simulink model "FDIA_21_TRAINING"  (R2021a)
settings: Solver=ode113  StartTime=0.0  StopTime=20  RelTol=1e-3
undefined symbols (not defined in the file or in its folder): Discrete, linsys1, Time
libraries: spsThreePhaseVIMeasurementLib x46, spsThreePhasePISectionLineLib x20, spsThreePhaseSeriesRLCLoadLib x12, simulink x6, spsThreePhaseTransformerTwoWindingsLib x5, spsThreePhaseBreakerLib x5, ctrlSharedLib x3, spsThreePhaseDynamicLoadLib x3, spsSynchronousMachinepuStandardLib x3, spsThreePhaseParallelRLCLoadLib x3, spsExcitationSystemLib x3, spsGenericPowerSystemStabilizerLib x3
(part 3 of 3)

== system FDIA_21_TRAINING/Subsystem1/Bus_1 ==
  Three-Phase V-I Measurement : spsThreePhaseVIMeasurementLib/Three-Phase V-I Measurement  VoltageMeasurement=phase-to-phase  SetLabelV=on  LabelV=VB_1  Vpu=off  VpuLL=off  CurrentMeasurement=yes  SetLabelI=on  LabelI=IB_1  Ipu=off  Pbase=100e6  Vbase=500e3  OutputType=Complex  PhasorSimulation=off  PSBequivalent=0
  Three-Phase V-I Measurement1 : spsThreePhaseVIMeasurementLib/Three-Phase V-I Measurement  VoltageMeasurement=phase-to-phase  SetLabelV=on  LabelV=V_B1  Vpu=off  VpuLL=off  CurrentMeasurement=yes  SetLabelI=on  LabelI=I_B1  Ipu=off  Pbase=100e6  Vbase=500e3  OutputType=Complex  PhasorSimulation=off  PSBequivalent=0
  Conn1 : PMIOPort  Side=Left
  Conn2 : PMIOPort  Port=2  Side=Right
  Conn3 : PMIOPort  Port=3  Side=Left
  Conn4 : PMIOPort  Port=4  Side=Right
  Conn5 : PMIOPort  Port=5  Side=Right
  Conn6 : PMIOPort  Port=6  Side=Left
  Conn7 : PMIOPort  Port=7  Side=Right
  Conn8 : PMIOPort  Port=8  Side=Right
  Conn9 : PMIOPort  Port=9  Side=Right
  connections:
  Conn6/RConn1 -- Three-Phase V-I Measurement1/LConn1 -- Three-Phase V-I Measurement/LConn3
  Three-Phase V-I Measurement/RConn2 -- Conn4/RConn1
  Three-Phase V-I Measurement1/RConn2 -- Conn8/RConn1
  Conn3/RConn1 -- Three-Phase V-I Measurement1/LConn2 -- Three-Phase V-I Measurement/LConn2
  Conn1/RConn1 -- Three-Phase V-I Measurement1/LConn3 -- Three-Phase V-I Measurement/LConn1
  Three-Phase V-I Measurement/RConn1 -- Conn5/RConn1
  Three-Phase V-I Measurement/RConn3 -- Conn2/RConn1
  Three-Phase V-I Measurement1/RConn1 -- Conn9/RConn1
  Three-Phase V-I Measurement1/RConn3 -- Conn7/RConn1

== system FDIA_21_TRAINING/Subsystem1/Bus_10 ==
  Three-Phase V-I Measurement : spsThreePhaseVIMeasurementLib/Three-Phase V-I Measurement  VoltageMeasurement=phase-to-phase  SetLabelV=on  LabelV=VB_10  Vpu=off  VpuLL=off  CurrentMeasurement=yes  SetLabelI=on  LabelI=IB_10  Ipu=off  Pbase=100e6  Vbase=500e3  OutputType=Complex  PhasorSimulation=off  PSBequivalent=0
  Three-Phase V-I Measurement1 : spsThreePhaseVIMeasurementLib/Three-Phase V-I Measurement  VoltageMeasurement=phase-to-phase  SetLabelV=on  LabelV=V_B10  Vpu=off  VpuLL=off  CurrentMeasurement=yes  SetLabelI=on  LabelI=I_B10  Ipu=off  Pbase=100e6  Vbase=500e3  OutputType=Complex  PhasorSimulation=off  PSBequivalent=0
  Conn1 : PMIOPort  Side=Left
  Conn2 : PMIOPort  Port=2  Side=Right
  Conn3 : PMIOPort  Port=3  Side=Left
  Conn4 : PMIOPort  Port=4  Side=Right
  Conn5 : PMIOPort  Port=5  Side=Right
  Conn6 : PMIOPort  Port=6  Side=Left
  Conn7 : PMIOPort  Port=7  Side=Right
  Conn8 : PMIOPort  Port=8  Side=Right
  Conn9 : PMIOPort  Port=9  Side=Right
  connections:
  Conn1/RConn1 -- Three-Phase V-I Measurement1/LConn3 -- Three-Phase V-I Measurement/LConn1
  Conn3/RConn1 -- Three-Phase V-I Measurement1/LConn2 -- Three-Phase V-I Measurement/LConn2
  Conn8/RConn1 -- Three-Phase V-I Measurement1/RConn2
  Three-Phase V-I Measurement/RConn2 -- Conn4/RConn1
  Conn6/RConn1 -- Three-Phase V-I Measurement1/LConn1 -- Three-Phase V-I Measurement/LConn3
  Conn7/RConn1 -- Three-Phase V-I Measurement1/RConn1
  Conn9/RConn1 -- Three-Phase V-I Measurement1/RConn3
  Conn2/RConn1 -- Three-Phase V-I Measurement/RConn1
  Conn5/RConn1 -- Three-Phase V-I Measurement/RConn3

== system FDIA_21_TRAINING/Subsystem1/Bus_11 ==
  Three-Phase V-I Measurement : spsThreePhaseVIMeasurementLib/Three-Phase V-I Measurement  VoltageMeasurement=phase-to-phase  SetLabelV=on  LabelV=VB_11  Vpu=off  VpuLL=off  CurrentMeasurement=yes  SetLabelI=on  LabelI=IB_11  Ipu=off  Pbase=100e6  Vbase=500e3  OutputType=Complex  PhasorSimulation=off  PSBequivalent=0
  Three-Phase V-I Measurement1 : spsThreePhaseVIMeasurementLib/Three-Phase V-I Measurement  VoltageMeasurement=phase-to-phase  SetLabelV=on  LabelV=V_B11  Vpu=off  VpuLL=off  CurrentMeasurement=yes  SetLabelI=on  LabelI=I_B11  Ipu=off  Pbase=100e6  Vbase=500e3  OutputType=Complex  PhasorSimulation=off  PSBequivalent=0
  Conn1 : PMIOPort  Side=Left
  Conn2 : PMIOPort  Port=2  Side=Right
  Conn3 : PMIOPort  Port=3  Side=Left
  Conn4 : PMIOPort  Port=4  Side=Right
  Conn5 : PMIOPort  Port=5  Side=Right
  Conn6 : PMIOPort  Port=6  Side=Left
  Conn7 : PMIOPort  Port=7  Side=Right
  Conn8 : PMIOPort  Port=8  Side=Right
  Conn9 : PMIOPort  Port=9  Side=Right
  connections:
  Three-Phase V-I Measurement/RConn3 -- Conn5/RConn1
  Three-Phase V-I Measurement/RConn1 -- Conn2/RConn1
  Three-Phase V-I Measurement1/RConn3 -- Conn9/RConn1
  Three-Phase V-I Measurement1/RConn1 -- Conn7/RConn1
  Conn6/RConn1 -- Three-Phase V-I Measurement1/LConn1 -- Three-Phase V-I Measurement/LConn3
  Three-Phase V-I Measurement/RConn2 -- Conn4/RConn1
  Three-Phase V-I Measurement1/RConn2 -- Conn8/RConn1
  Conn3/RConn1 -- Three-Phase V-I Measurement1/LConn2 -- Three-Phase V-I Measurement/LConn2
  Conn1/RConn1 -- Three-Phase V-I Measurement1/LConn3 -- Three-Phase V-I Measurement/LConn1

== system FDIA_21_TRAINING/Subsystem1/Bus_12 ==
  Three-Phase V-I Measurement : spsThreePhaseVIMeasurementLib/Three-Phase V-I Measurement  VoltageMeasurement=phase-to-phase  SetLabelV=on  LabelV=VB_12  Vpu=off  VpuLL=off  CurrentMeasurement=yes  SetLabelI=on  LabelI=IB_12  Ipu=off  Pbase=100e6  Vbase=500e3  OutputType=Complex  PhasorSimulation=off  PSBequivalent=0
  Three-Phase V-I Measurement1 : spsThreePhaseVIMeasurementLib/Three-Phase V-I Measurement  VoltageMeasurement=phase-to-phase  SetLabelV=on  LabelV=V_B12  Vpu=off  VpuLL=off  CurrentMeasurement=yes  SetLabelI=on  LabelI=I_B12  Ipu=off  Pbase=100e6  Vbase=500e3  OutputType=Complex  PhasorSimulation=off  PSBequivalent=0
  Conn1 : PMIOPort  Side=Left
  Conn2 : PMIOPort  Port=2  Side=Right
  Conn3 : PMIOPort  Port=3  Side=Left
  Conn4 : PMIOPort  Port=4  Side=Right
  Conn5 : PMIOPort  Port=5  Side=Right
  Conn6 : PMIOPort  Port=6  Side=Left
  Conn7 : PMIOPort  Port=7  Side=Right
  Conn8 : PMIOPort  Port=8  Side=Right
  Conn9 : PMIOPort  Port=9  Side=Right
  connections:
  Conn1/RConn1 -- Three-Phase V-I Measurement1/LConn3 -- Three-Phase V-I Measurement/LConn1
  Conn3/RConn1 -- Three-Phase V-I Measurement1/LConn2 -- Three-Phase V-I Measurement/LConn2
  Three-Phase V-I Measurement1/RConn2 -- Conn8/RConn1
  Conn4/RConn1 -- Three-Phase V-I Measurement/RConn2
  Conn6/RConn1 -- Three-Phase V-I Measurement1/LConn1 -- Three-Phase V-I Measurement/LConn3
  Three-Phase V-I Measurement1/RConn1 -- Conn7/RConn1
  Three-Phase V-I Measurement1/RConn3 -- Conn9/RConn1
  Conn2/RConn1 -- Three-Phase V-I Measurement/RConn1
  Conn5/RConn1 -- Three-Phase V-I Measurement/RConn3

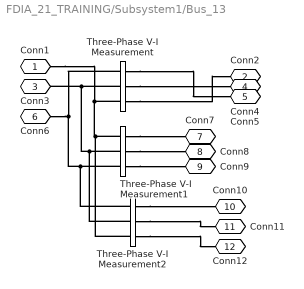
== system FDIA_21_TRAINING/Subsystem1/Bus_13 ==
  Three-Phase V-I Measurement : spsThreePhaseVIMeasurementLib/Three-Phase V-I Measurement  VoltageMeasurement=phase-to-phase  SetLabelV=on  LabelV=VB_13  Vpu=off  VpuLL=off  CurrentMeasurement=yes  SetLabelI=on  LabelI=IB_13  Ipu=off  Pbase=100e6  Vbase=500e3  OutputType=Complex  PhasorSimulation=off  PSBequivalent=0
  Three-Phase V-I Measurement1 : spsThreePhaseVIMeasurementLib/Three-Phase V-I Measurement  VoltageMeasurement=phase-to-phase  SetLabelV=on  LabelV=V_B13_13  Vpu=off  VpuLL=off  CurrentMeasurement=yes  SetLabelI=on  LabelI=I_B13_13  Ipu=off  Pbase=100e6  Vbase=500e3  OutputType=Complex  PhasorSimulation=off  PSBequivalent=0
  Three-Phase V-I Measurement2 : spsThreePhaseVIMeasurementLib/Three-Phase V-I Measurement  VoltageMeasurement=phase-to-phase  SetLabelV=on  LabelV=V_B13  Vpu=off  VpuLL=off  CurrentMeasurement=yes  SetLabelI=on  LabelI=I_B13  Ipu=off  Pbase=100e6  Vbase=500e3  OutputType=Complex  PhasorSimulation=off  PSBequivalent=0
  Conn1 : PMIOPort  Side=Left
  Conn2 : PMIOPort  Port=2  Side=Right
  Conn3 : PMIOPort  Port=3  Side=Left
  Conn4 : PMIOPort  Port=4  Side=Right
  Conn5 : PMIOPort  Port=5  Side=Right
  Conn6 : PMIOPort  Port=6  Side=Left
  Conn7 : PMIOPort  Port=7  Side=Right
  Conn8 : PMIOPort  Port=8  Side=Right
  Conn9 : PMIOPort  Port=9  Side=Right
  Conn10 : PMIOPort  Port=10  Side=Right
  Conn11 : PMIOPort  Port=11  Side=Right
  Conn12 : PMIOPort  Port=12  Side=Right
  connections:
  Three-Phase V-I Measurement2/LConn1 -- Three-Phase V-I Measurement1/LConn3 -- Three-Phase V-I Measurement/LConn1 -- Conn6/RConn1
  Conn3/RConn1 -- Three-Phase V-I Measurement/LConn2 -- Three-Phase V-I Measurement2/LConn2 -- Three-Phase V-I Measurement1/LConn2
  Three-Phase V-I Measurement1/RConn2 -- Conn8/RConn1
  Three-Phase V-I Measurement/RConn2 -- Conn4/RConn1
  Three-Phase V-I Measurement2/LConn3 -- Three-Phase V-I Measurement1/LConn1 -- Three-Phase V-I Measurement/LConn3 -- Conn1/RConn1
  Three-Phase V-I Measurement1/RConn1 -- Conn7/RConn1
  Three-Phase V-I Measurement1/RConn3 -- Conn9/RConn1
  Three-Phase V-I Measurement2/RConn1 -- Conn10/RConn1
  Three-Phase V-I Measurement2/RConn2 -- Conn11/RConn1
  Three-Phase V-I Measurement2/RConn3 -- Conn12/RConn1
  Three-Phase V-I Measurement/RConn1 -- Conn5/RConn1
  Three-Phase V-I Measurement/RConn3 -- Conn2/RConn1

== system FDIA_21_TRAINING/Subsystem1/Bus_14 ==
  Three-Phase V-I Measurement : spsThreePhaseVIMeasurementLib/Three-Phase V-I Measurement  VoltageMeasurement=phase-to-phase  SetLabelV=on  LabelV=VB_14  Vpu=off  VpuLL=off  CurrentMeasurement=yes  SetLabelI=on  LabelI=IB_14  Ipu=off  Pbase=100e6  Vbase=500e3  OutputType=Complex  PhasorSimulation=off  PSBequivalent=0
  Three-Phase V-I Measurement1 : spsThreePhaseVIMeasurementLib/Three-Phase V-I Measurement  VoltageMeasurement=phase-to-phase  SetLabelV=on  LabelV=V_B14  Vpu=off  VpuLL=off  CurrentMeasurement=yes  SetLabelI=on  LabelI=I_B14  Ipu=off  Pbase=100e6  Vbase=500e3  OutputType=Complex  PhasorSimulation=off  PSBequivalent=0
  Conn1 : PMIOPort  Side=Left
  Conn2 : PMIOPort  Port=2  Side=Right
  Conn3 : PMIOPort  Port=3  Side=Left
  Conn4 : PMIOPort  Port=4  Side=Right
  Conn5 : PMIOPort  Port=5  Side=Right
  Conn6 : PMIOPort  Port=6  Side=Left
  Conn7 : PMIOPort  Port=7  Side=Right
  Conn8 : PMIOPort  Port=8  Side=Right
  Conn9 : PMIOPort  Port=9  Side=Right
  connections:
  Conn1/RConn1 -- Three-Phase V-I Measurement1/LConn3 -- Three-Phase V-I Measurement/LConn1
  Conn3/RConn1 -- Three-Phase V-I Measurement1/LConn2 -- Three-Phase V-I Measurement/LConn2
  Three-Phase V-I Measurement1/RConn2 -- Conn8/RConn1
  Three-Phase V-I Measurement/RConn2 -- Conn4/RConn1
  Conn6/RConn1 -- Three-Phase V-I Measurement1/LConn1 -- Three-Phase V-I Measurement/LConn3
  Three-Phase V-I Measurement/RConn1 -- Conn2/RConn1
  Three-Phase V-I Measurement/RConn3 -- Conn5/RConn1
  Three-Phase V-I Measurement1/RConn3 -- Conn7/RConn1
  Three-Phase V-I Measurement1/RConn1 -- Conn9/RConn1

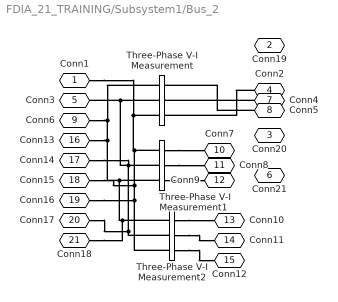
== system FDIA_21_TRAINING/Subsystem1/Bus_2 ==
  Three-Phase V-I Measurement : spsThreePhaseVIMeasurementLib/Three-Phase V-I Measurement  VoltageMeasurement=phase-to-phase  SetLabelV=on  LabelV=VB_2  Vpu=off  VpuLL=off  CurrentMeasurement=yes  SetLabelI=on  LabelI=IB_2  Ipu=off  Pbase=100e6  Vbase=500e3  OutputType=Complex  PhasorSimulation=off  PSBequivalent=0
  Three-Phase V-I Measurement1 : spsThreePhaseVIMeasurementLib/Three-Phase V-I Measurement  VoltageMeasurement=phase-to-phase  SetLabelV=on  LabelV=V_B22  Vpu=off  VpuLL=off  CurrentMeasurement=yes  SetLabelI=on  LabelI=I_B22  Ipu=off  Pbase=100e6  Vbase=500e3  OutputType=Complex  PhasorSimulation=off  PSBequivalent=0
  Three-Phase V-I Measurement2 : spsThreePhaseVIMeasurementLib/Three-Phase V-I Measurement  VoltageMeasurement=phase-to-phase  SetLabelV=on  LabelV=V_B2  Vpu=off  VpuLL=off  CurrentMeasurement=yes  SetLabelI=on  LabelI=I_B2  Ipu=off  Pbase=100e6  Vbase=500e3  OutputType=Complex  PhasorSimulation=off  PSBequivalent=0
  Conn1 : PMIOPort  Side=Left
  Conn19 : PMIOPort  Port=2  Side=Right
  Conn20 : PMIOPort  Port=3  Side=Right
  Conn2 : PMIOPort  Port=4  Side=Right
  Conn3 : PMIOPort  Port=5  Side=Left
  Conn21 : PMIOPort  Port=6  Side=Right
  Conn4 : PMIOPort  Port=7  Side=Right
  Conn5 : PMIOPort  Port=8  Side=Right
  Conn6 : PMIOPort  Port=9  Side=Left
  Conn7 : PMIOPort  Port=10  Side=Right
  Conn8 : PMIOPort  Port=11  Side=Right
  Conn9 : PMIOPort  Port=12  Side=Right
  Conn10 : PMIOPort  Port=13  Side=Right
  Conn11 : PMIOPort  Port=14  Side=Right
  Conn12 : PMIOPort  Port=15  Side=Right
  Conn13 : PMIOPort  Port=16  Side=Left
  Conn14 : PMIOPort  Port=17  Side=Left
  Conn15 : PMIOPort  Port=18  Side=Left
  Conn16 : PMIOPort  Port=19  Side=Left
  Conn17 : PMIOPort  Port=20  Side=Left
  Conn18 : PMIOPort  Port=21  Side=Left
  connections:
  Conn18/RConn1 -- Three-Phase V-I Measurement2/LConn1 -- Three-Phase V-I Measurement1/LConn3 -- Conn13/RConn1 -- Three-Phase V-I Measurement/LConn1 -- Conn6/RConn1
  Conn3/RConn1 -- Three-Phase V-I Measurement/LConn2 -- Three-Phase V-I Measurement1/LConn2 -- Three-Phase V-I Measurement2/LConn2 -- Conn17/RConn1 -- Conn14/RConn1
  Three-Phase V-I Measurement1/RConn2 -- Conn8/RConn1
  Conn4/RConn1 -- Three-Phase V-I Measurement/RConn2
  Conn16/RConn1 -- Three-Phase V-I Measurement2/LConn3 -- Conn15/RConn1 -- Three-Phase V-I Measurement1/LConn1 -- Three-Phase V-I Measurement/LConn3 -- Conn1/RConn1
  Three-Phase V-I Measurement1/RConn1 -- Conn7/RConn1
  Three-Phase V-I Measurement1/RConn3 -- Conn9/RConn1
  Three-Phase V-I Measurement2/RConn1 -- Conn10/RConn1
  Three-Phase V-I Measurement2/RConn2 -- Conn11/RConn1
  Three-Phase V-I Measurement2/RConn3 -- Conn12/RConn1
  Conn5/RConn1 -- Three-Phase V-I Measurement/RConn1
  Conn2/RConn1 -- Three-Phase V-I Measurement/RConn3

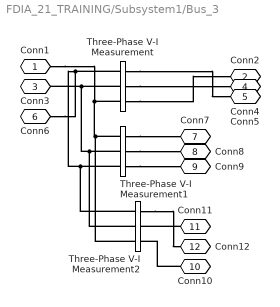
== system FDIA_21_TRAINING/Subsystem1/Bus_3 ==
  Three-Phase V-I Measurement : spsThreePhaseVIMeasurementLib/Three-Phase V-I Measurement  VoltageMeasurement=phase-to-phase  SetLabelV=on  LabelV=VB_3  Vpu=off  VpuLL=off  CurrentMeasurement=yes  SetLabelI=on  LabelI=IB_3  Ipu=off  Pbase=100e6  Vbase=500e3  OutputType=Complex  PhasorSimulation=off  PSBequivalent=0
  Three-Phase V-I Measurement1 : spsThreePhaseVIMeasurementLib/Three-Phase V-I Measurement  VoltageMeasurement=phase-to-phase  SetLabelV=on  LabelV=V_B33  Vpu=off  VpuLL=off  CurrentMeasurement=yes  SetLabelI=on  LabelI=I_B33  Ipu=off  Pbase=100e6  Vbase=500e3  OutputType=Complex  PhasorSimulation=off  PSBequivalent=0
  Three-Phase V-I Measurement2 : spsThreePhaseVIMeasurementLib/Three-Phase V-I Measurement  VoltageMeasurement=phase-to-phase  SetLabelV=on  LabelV=V_B3  Vpu=off  VpuLL=off  CurrentMeasurement=yes  SetLabelI=on  LabelI=I_B3  Ipu=off  Pbase=100e6  Vbase=500e3  OutputType=Complex  PhasorSimulation=off  PSBequivalent=0
  Conn1 : PMIOPort  Side=Left
  Conn2 : PMIOPort  Port=2  Side=Right
  Conn3 : PMIOPort  Port=3  Side=Left
  Conn4 : PMIOPort  Port=4  Side=Right
  Conn5 : PMIOPort  Port=5  Side=Right
  Conn6 : PMIOPort  Port=6  Side=Left
  Conn7 : PMIOPort  Port=7  Side=Right
  Conn8 : PMIOPort  Port=8  Side=Right
  Conn9 : PMIOPort  Port=9  Side=Right
  Conn10 : PMIOPort  Port=10  Side=Right
  Conn11 : PMIOPort  Port=11  Side=Right
  Conn12 : PMIOPort  Port=12  Side=Right
  connections:
  Conn11/RConn1 -- Three-Phase V-I Measurement2/RConn2
  Three-Phase V-I Measurement1/RConn3 -- Conn9/RConn1
  Three-Phase V-I Measurement1/RConn1 -- Conn7/RConn1
  Three-Phase V-I Measurement2/LConn3 -- Three-Phase V-I Measurement1/LConn1 -- Three-Phase V-I Measurement/LConn3 -- Conn1/RConn1
  Three-Phase V-I Measurement/RConn2 -- Conn4/RConn1
  Three-Phase V-I Measurement1/RConn2 -- Conn8/RConn1
  Three-Phase V-I Measurement2/LConn2 -- Three-Phase V-I Measurement1/LConn2 -- Three-Phase V-I Measurement/LConn2 -- Conn3/RConn1
  Three-Phase V-I Measurement2/LConn1 -- Three-Phase V-I Measurement1/LConn3 -- Three-Phase V-I Measurement/LConn1 -- Conn6/RConn1
  Conn10/RConn1 -- Three-Phase V-I Measurement2/RConn3
  Three-Phase V-I Measurement2/RConn1 -- Conn12/RConn1
  Three-Phase V-I Measurement/RConn3 -- Conn2/RConn1
  Three-Phase V-I Measurement/RConn1 -- Conn5/RConn1

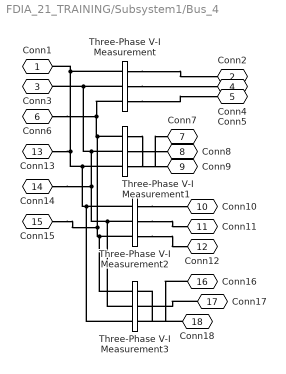
== system FDIA_21_TRAINING/Subsystem1/Bus_4 ==
  Three-Phase V-I Measurement : spsThreePhaseVIMeasurementLib/Three-Phase V-I Measurement  VoltageMeasurement=phase-to-phase  SetLabelV=on  LabelV=VB_4  Vpu=off  VpuLL=off  CurrentMeasurement=yes  SetLabelI=on  LabelI=IB_4  Ipu=off  Pbase=100e6  Vbase=500e3  OutputType=Complex  PhasorSimulation=off  PSBequivalent=0
  Three-Phase V-I Measurement1 : spsThreePhaseVIMeasurementLib/Three-Phase V-I Measurement  VoltageMeasurement=phase-to-phase  SetLabelV=on  LabelV=V_B44  Vpu=off  VpuLL=off  CurrentMeasurement=yes  SetLabelI=on  LabelI=I_B44  Ipu=off  Pbase=100e6  Vbase=500e3  OutputType=Complex  PhasorSimulation=off  PSBequivalent=0
  Three-Phase V-I Measurement2 : spsThreePhaseVIMeasurementLib/Three-Phase V-I Measurement  VoltageMeasurement=phase-to-phase  SetLabelV=on  LabelV=V_B4  Vpu=off  VpuLL=off  CurrentMeasurement=yes  SetLabelI=on  LabelI=I_B4  Ipu=off  Pbase=100e6  Vbase=500e3  OutputType=Complex  PhasorSimulation=off  PSBequivalent=0
  Three-Phase V-I Measurement3 : spsThreePhaseVIMeasurementLib/Three-Phase V-I Measurement  VoltageMeasurement=phase-to-phase  SetLabelV=on  LabelV=V_B4_4  Vpu=off  VpuLL=off  CurrentMeasurement=yes  SetLabelI=on  LabelI=I_B4_4  Ipu=off  Pbase=100e6  Vbase=500e3  OutputType=Complex  PhasorSimulation=off  PSBequivalent=0
  Conn1 : PMIOPort  Side=Left
  Conn2 : PMIOPort  Port=2  Side=Right
  Conn3 : PMIOPort  Port=3  Side=Left
  Conn4 : PMIOPort  Port=4  Side=Right
  Conn5 : PMIOPort  Port=5  Side=Right
  Conn6 : PMIOPort  Port=6  Side=Left
  Conn7 : PMIOPort  Port=7  Side=Right
  Conn8 : PMIOPort  Port=8  Side=Right
  Conn9 : PMIOPort  Port=9  Side=Right
  Conn10 : PMIOPort  Port=10  Side=Right
  Conn11 : PMIOPort  Port=11  Side=Right
  Conn12 : PMIOPort  Port=12  Side=Right
  Conn13 : PMIOPort  Port=13  Side=Left
  Conn14 : PMIOPort  Port=14  Side=Left
  Conn15 : PMIOPort  Port=15  Side=Left
  Conn16 : PMIOPort  Port=16  Side=Right
  Conn17 : PMIOPort  Port=17  Side=Right
  Conn18 : PMIOPort  Port=18  Side=Right
  connections:
  Conn1/RConn1 -- Three-Phase V-I Measurement/LConn1 -- Three-Phase V-I Measurement1/LConn3 -- Three-Phase V-I Measurement3/LConn3 -- Three-Phase V-I Measurement2/LConn1 -- Conn13/RConn1
  Conn3/RConn1 -- Three-Phase V-I Measurement/LConn2 -- Three-Phase V-I Measurement1/LConn2 -- Three-Phase V-I Measurement3/LConn2 -- Three-Phase V-I Measurement2/LConn2 -- Conn14/RConn1
  Three-Phase V-I Measurement1/RConn2 -- Conn8/RConn1
  Three-Phase V-I Measurement/RConn2 -- Conn4/RConn1
  Conn6/RConn1 -- Three-Phase V-I Measurement/LConn3 -- Three-Phase V-I Measurement1/LConn1 -- Three-Phase V-I Measurement3/LConn1 -- Three-Phase V-I Measurement2/LConn3 -- Conn15/RConn1
  Three-Phase V-I Measurement2/RConn1 -- Conn10/RConn1
  Three-Phase V-I Measurement2/RConn2 -- Conn11/RConn1
  Three-Phase V-I Measurement2/RConn3 -- Conn12/RConn1
  Three-Phase V-I Measurement1/RConn1 -- Conn9/RConn1
  Three-Phase V-I Measurement1/RConn3 -- Conn7/RConn1
  Three-Phase V-I Measurement/RConn3 -- Conn5/RConn1
  Three-Phase V-I Measurement/RConn1 -- Conn2/RConn1
  Conn17/RConn1 -- Three-Phase V-I Measurement3/RConn2
  Conn16/RConn1 -- Three-Phase V-I Measurement3/RConn3
  Conn18/RConn1 -- Three-Phase V-I Measurement3/RConn1

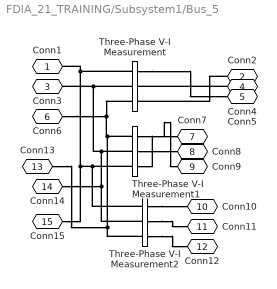
== system FDIA_21_TRAINING/Subsystem1/Bus_5 ==
  Three-Phase V-I Measurement : spsThreePhaseVIMeasurementLib/Three-Phase V-I Measurement  VoltageMeasurement=phase-to-phase  SetLabelV=on  LabelV=VB_5  Vpu=off  VpuLL=off  CurrentMeasurement=yes  SetLabelI=on  LabelI=IB_5  Ipu=off  Pbase=100e6  Vbase=500e3  OutputType=Complex  PhasorSimulation=off  PSBequivalent=0
  Three-Phase V-I Measurement1 : spsThreePhaseVIMeasurementLib/Three-Phase V-I Measurement  VoltageMeasurement=phase-to-phase  SetLabelV=on  LabelV=V_B55  Vpu=off  VpuLL=off  CurrentMeasurement=yes  SetLabelI=on  LabelI=I_B55  Ipu=off  Pbase=100e6  Vbase=500e3  OutputType=Complex  PhasorSimulation=off  PSBequivalent=0
  Three-Phase V-I Measurement2 : spsThreePhaseVIMeasurementLib/Three-Phase V-I Measurement  VoltageMeasurement=phase-to-phase  SetLabelV=on  LabelV=V_B5  Vpu=off  VpuLL=off  CurrentMeasurement=yes  SetLabelI=on  LabelI=I_B5  Ipu=off  Pbase=100e6  Vbase=500e3  OutputType=Complex  PhasorSimulation=off  PSBequivalent=0
  Conn1 : PMIOPort  Side=Left
  Conn2 : PMIOPort  Port=2  Side=Right
  Conn3 : PMIOPort  Port=3  Side=Left
  Conn4 : PMIOPort  Port=4  Side=Right
  Conn5 : PMIOPort  Port=5  Side=Right
  Conn6 : PMIOPort  Port=6  Side=Left
  Conn7 : PMIOPort  Port=7  Side=Right
  Conn8 : PMIOPort  Port=8  Side=Right
  Conn9 : PMIOPort  Port=9  Side=Right
  Conn10 : PMIOPort  Port=10  Side=Right
  Conn11 : PMIOPort  Port=11  Side=Right
  Conn12 : PMIOPort  Port=12  Side=Right
  Conn13 : PMIOPort  Port=13  Side=Left
  Conn14 : PMIOPort  Port=14  Side=Left
  Conn15 : PMIOPort  Port=15  Side=Left
  connections:
  Three-Phase V-I Measurement2/RConn3 -- Conn12/RConn1
  Three-Phase V-I Measurement2/RConn2 -- Conn11/RConn1
  Three-Phase V-I Measurement2/RConn1 -- Conn10/RConn1
  Conn13/RConn1 -- Three-Phase V-I Measurement2/LConn3 -- Three-Phase V-I Measurement1/LConn1 -- Three-Phase V-I Measurement/LConn3 -- Conn6/RConn1
  Conn4/RConn1 -- Three-Phase V-I Measurement/RConn2
  Three-Phase V-I Measurement1/RConn2 -- Conn8/RConn1
  Conn14/RConn1 -- Three-Phase V-I Measurement2/LConn2 -- Three-Phase V-I Measurement1/LConn2 -- Three-Phase V-I Measurement/LConn2 -- Conn3/RConn1
  Three-Phase V-I Measurement2/LConn1 -- Three-Phase V-I Measurement1/LConn3 -- Three-Phase V-I Measurement/LConn1 -- Conn1/RConn1 -- Conn15/RConn1
  Three-Phase V-I Measurement1/RConn3 -- Conn7/RConn1
  Three-Phase V-I Measurement1/RConn1 -- Conn9/RConn1
  Three-Phase V-I Measurement/RConn1 -- Conn5/RConn1
  Conn2/RConn1 -- Three-Phase V-I Measurement/RConn3

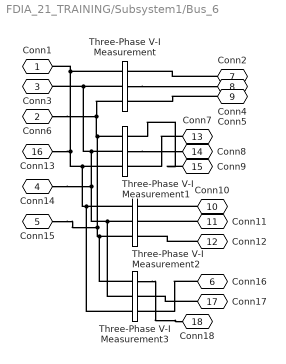
== system FDIA_21_TRAINING/Subsystem1/Bus_6 ==
  Three-Phase V-I Measurement : spsThreePhaseVIMeasurementLib/Three-Phase V-I Measurement  VoltageMeasurement=phase-to-phase  SetLabelV=on  LabelV=VB_6  Vpu=off  VpuLL=off  CurrentMeasurement=yes  SetLabelI=on  LabelI=IB_6  Ipu=off  Pbase=100e6  Vbase=500e3  OutputType=Complex  PhasorSimulation=off  PSBequivalent=0
  Three-Phase V-I Measurement1 : spsThreePhaseVIMeasurementLib/Three-Phase V-I Measurement  VoltageMeasurement=phase-to-phase  SetLabelV=on  LabelV=V_B66  Vpu=off  VpuLL=off  CurrentMeasurement=yes  SetLabelI=on  LabelI=I_B66  Ipu=off  Pbase=100e6  Vbase=500e3  OutputType=Complex  PhasorSimulation=off  PSBequivalent=0
  Three-Phase V-I Measurement2 : spsThreePhaseVIMeasurementLib/Three-Phase V-I Measurement  VoltageMeasurement=phase-to-phase  SetLabelV=on  LabelV=V_B6  Vpu=off  VpuLL=off  CurrentMeasurement=yes  SetLabelI=on  LabelI=I_B6  Ipu=off  Pbase=100e6  Vbase=500e3  OutputType=Complex  PhasorSimulation=off  PSBequivalent=0
  Three-Phase V-I Measurement3 : spsThreePhaseVIMeasurementLib/Three-Phase V-I Measurement  VoltageMeasurement=phase-to-phase  SetLabelV=on  LabelV=V_B6_6  Vpu=off  VpuLL=off  CurrentMeasurement=yes  SetLabelI=on  LabelI=I_B6_6  Ipu=off  Pbase=100e6  Vbase=500e3  OutputType=Complex  PhasorSimulation=off  PSBequivalent=0
  Conn1 : PMIOPort  Side=Left
  Conn6 : PMIOPort  Port=2  Side=Left
  Conn3 : PMIOPort  Port=3  Side=Left
  Conn14 : PMIOPort  Port=4  Side=Left
  Conn15 : PMIOPort  Port=5  Side=Left
  Conn16 : PMIOPort  Port=6  Side=Right
  Conn2 : PMIOPort  Port=7  Side=Right
  Conn4 : PMIOPort  Port=8  Side=Right
  Conn5 : PMIOPort  Port=9  Side=Right
  Conn10 : PMIOPort  Port=10  Side=Right
  Conn11 : PMIOPort  Port=11  Side=Right
  Conn12 : PMIOPort  Port=12  Side=Right
  Conn7 : PMIOPort  Port=13  Side=Right
  Conn8 : PMIOPort  Port=14  Side=Right
  Conn9 : PMIOPort  Port=15  Side=Right
  Conn13 : PMIOPort  Port=16  Side=Right
  Conn17 : PMIOPort  Port=17  Side=Right
  Conn18 : PMIOPort  Port=18  Side=Right
  connections:
  Conn17/RConn1 -- Three-Phase V-I Measurement3/RConn2
  Conn12/RConn1 -- Three-Phase V-I Measurement2/RConn3
  Conn11/RConn1 -- Three-Phase V-I Measurement2/RConn2
  Conn10/RConn1 -- Three-Phase V-I Measurement2/RConn1
  Conn5/RConn1 -- Three-Phase V-I Measurement/RConn3
  Conn2/RConn1 -- Three-Phase V-I Measurement/RConn1
  Three-Phase V-I Measurement3/LConn1 -- Three-Phase V-I Measurement2/LConn3 -- Conn15/RConn1 -- Three-Phase V-I Measurement1/LConn1 -- Three-Phase V-I Measurement/LConn3 -- Conn6/RConn1
  Three-Phase V-I Measurement/RConn2 -- Conn4/RConn1
  Three-Phase V-I Measurement1/RConn2 -- Conn8/RConn1
  Three-Phase V-I Measurement3/LConn2 -- Three-Phase V-I Measurement2/LConn2 -- Conn14/RConn1 -- Three-Phase V-I Measurement1/LConn2 -- Three-Phase V-I Measurement/LConn2 -- Conn3/RConn1
  Three-Phase V-I Measurement3/LConn3 -- Three-Phase V-I Measurement2/LConn1 -- Three-Phase V-I Measurement1/LConn3 -- Conn13/RConn1 -- Three-Phase V-I Measurement/LConn1 -- Conn1/RConn1
  Conn7/RConn1 -- Three-Phase V-I Measurement1/RConn3
  Conn9/RConn1 -- Three-Phase V-I Measurement1/RConn1
  Conn16/RConn1 -- Three-Phase V-I Measurement3/RConn3
  Three-Phase V-I Measurement3/RConn1 -- Conn18/RConn1

== system FDIA_21_TRAINING/Subsystem1/Bus_7 ==
  Three-Phase V-I Measurement : spsThreePhaseVIMeasurementLib/Three-Phase V-I Measurement  VoltageMeasurement=phase-to-phase  SetLabelV=on  LabelV=VB_7  Vpu=off  VpuLL=off  CurrentMeasurement=yes  SetLabelI=on  LabelI=IB_7  Ipu=off  Pbase=100e6  Vbase=500e3  OutputType=Complex  PhasorSimulation=off  PSBequivalent=0
  Three-Phase V-I Measurement1 : spsThreePhaseVIMeasurementLib/Three-Phase V-I Measurement  VoltageMeasurement=phase-to-phase  SetLabelV=on  LabelV=V_B7  Vpu=off  VpuLL=off  CurrentMeasurement=yes  SetLabelI=on  LabelI=I_B7  Ipu=off  Pbase=100e6  Vbase=500e3  OutputType=Complex  PhasorSimulation=off  PSBequivalent=0
  Conn1 : PMIOPort  Side=Left
  Conn2 : PMIOPort  Port=2  Side=Right
  Conn3 : PMIOPort  Port=3  Side=Left
  Conn4 : PMIOPort  Port=4  Side=Right
  Conn5 : PMIOPort  Port=5  Side=Right
  Conn6 : PMIOPort  Port=6  Side=Left
  Conn7 : PMIOPort  Port=7  Side=Right
  Conn8 : PMIOPort  Port=8  Side=Right
  Conn9 : PMIOPort  Port=9  Side=Right
  connections:
  Conn6/RConn1 -- Three-Phase V-I Measurement1/LConn3 -- Three-Phase V-I Measurement/LConn1
  Conn3/RConn1 -- Three-Phase V-I Measurement1/LConn2 -- Three-Phase V-I Measurement/LConn2
  Conn8/RConn1 -- Three-Phase V-I Measurement1/RConn2
  Conn4/RConn1 -- Three-Phase V-I Measurement/RConn2
  Conn1/RConn1 -- Three-Phase V-I Measurement1/LConn1 -- Three-Phase V-I Measurement/LConn3
  Conn7/RConn1 -- Three-Phase V-I Measurement1/RConn1
  Conn9/RConn1 -- Three-Phase V-I Measurement1/RConn3
  Conn2/RConn1 -- Three-Phase V-I Measurement/RConn3
  Three-Phase V-I Measurement/RConn1 -- Conn5/RConn1

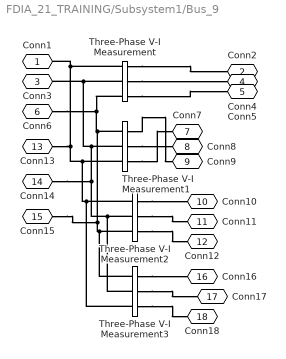
== system FDIA_21_TRAINING/Subsystem1/Bus_9 ==
  Three-Phase V-I Measurement : spsThreePhaseVIMeasurementLib/Three-Phase V-I Measurement  VoltageMeasurement=phase-to-phase  SetLabelV=on  LabelV=VB_9  Vpu=off  VpuLL=off  CurrentMeasurement=yes  SetLabelI=on  LabelI=IB_9  Ipu=off  Pbase=100e6  Vbase=500e3  OutputType=Complex  PhasorSimulation=off  PSBequivalent=0
  Three-Phase V-I Measurement1 : spsThreePhaseVIMeasurementLib/Three-Phase V-I Measurement  VoltageMeasurement=phase-to-phase  SetLabelV=on  LabelV=V_B9_9  Vpu=off  VpuLL=off  CurrentMeasurement=yes  SetLabelI=on  LabelI=I_B9_9  Ipu=off  Pbase=100e6  Vbase=500e3  OutputType=Complex  PhasorSimulation=off  PSBequivalent=0
  Three-Phase V-I Measurement2 : spsThreePhaseVIMeasurementLib/Three-Phase V-I Measurement  VoltageMeasurement=phase-to-phase  SetLabelV=on  LabelV=V_B9  Vpu=off  VpuLL=off  CurrentMeasurement=yes  SetLabelI=on  LabelI=I_B9  Ipu=off  Pbase=100e6  Vbase=500e3  OutputType=Complex  PhasorSimulation=off  PSBequivalent=0
  Three-Phase V-I Measurement3 : spsThreePhaseVIMeasurementLib/Three-Phase V-I Measurement  VoltageMeasurement=phase-to-phase  SetLabelV=on  LabelV=V_B9__9  Vpu=off  VpuLL=off  CurrentMeasurement=yes  SetLabelI=on  LabelI=I_B9__9  Ipu=off  Pbase=100e6  Vbase=500e3  OutputType=Complex  PhasorSimulation=off  PSBequivalent=0
  Conn1 : PMIOPort  Side=Left
  Conn2 : PMIOPort  Port=2  Side=Right
  Conn3 : PMIOPort  Port=3  Side=Left
  Conn4 : PMIOPort  Port=4  Side=Right
  Conn5 : PMIOPort  Port=5  Side=Right
  Conn6 : PMIOPort  Port=6  Side=Left
  Conn7 : PMIOPort  Port=7  Side=Right
  Conn8 : PMIOPort  Port=8  Side=Right
  Conn9 : PMIOPort  Port=9  Side=Right
  Conn10 : PMIOPort  Port=10  Side=Right
  Conn11 : PMIOPort  Port=11  Side=Right
  Conn12 : PMIOPort  Port=12  Side=Right
  Conn13 : PMIOPort  Port=13  Side=Left
  Conn14 : PMIOPort  Port=14  Side=Left
  Conn15 : PMIOPort  Port=15  Side=Left
  Conn16 : PMIOPort  Port=16  Side=Right
  Conn17 : PMIOPort  Port=17  Side=Right
  Conn18 : PMIOPort  Port=18  Side=Right
  connections:
  Conn1/RConn1 -- Three-Phase V-I Measurement/LConn1 -- Conn13/RConn1 -- Three-Phase V-I Measurement1/LConn3 -- Three-Phase V-I Measurement3/LConn3 -- Three-Phase V-I Measurement2/LConn1
  Conn3/RConn1 -- Three-Phase V-I Measurement/LConn2 -- Three-Phase V-I Measurement1/LConn2 -- Conn14/RConn1 -- Three-Phase V-I Measurement3/LConn2 -- Three-Phase V-I Measurement2/LConn2
  Three-Phase V-I Measurement1/RConn2 -- Conn8/RConn1
  Three-Phase V-I Measurement/RConn2 -- Conn4/RConn1
  Conn6/RConn1 -- Three-Phase V-I Measurement/LConn3 -- Three-Phase V-I Measurement1/LConn1 -- Conn15/RConn1 -- Three-Phase V-I Measurement3/LConn1 -- Three-Phase V-I Measurement2/LConn3
  Three-Phase V-I Measurement/RConn1 -- Conn2/RConn1
  Three-Phase V-I Measurement/RConn3 -- Conn5/RConn1
  Three-Phase V-I Measurement2/RConn1 -- Conn10/RConn1
  Three-Phase V-I Measurement2/RConn2 -- Conn11/RConn1
  Three-Phase V-I Measurement2/RConn3 -- Conn12/RConn1
  Three-Phase V-I Measurement3/RConn1 -- Conn16/RConn1
  Three-Phase V-I Measurement3/RConn2 -- Conn17/RConn1
  Three-Phase V-I Measurement3/RConn3 -- Conn18/RConn1
  Three-Phase V-I Measurement1/RConn3 -- Conn7/RConn1
  Three-Phase V-I Measurement1/RConn1 -- Conn9/RConn1

== system FDIA_21_TRAINING/Subsystem1/Power Flow Sensor 1 ==
  In1 : Inport
  In3 : Inport  Port=2
  In4 : Inport  Port=3
  Constant : Constant
  Matrix Multiply4 : Product  Multiplication=Matrix(*)
  Mux2 : Mux  Inputs=2
  Sum5 : Sum  Inputs=|++
  Three-Phase Dynamic Load2 : spsThreePhaseDynamicLoadLib/Three-Phase Dynamic Load  NominalVoltage="[ (217684)*1  60 ]"  ActiveReactivePowers=[11304000 0]  PositiveSequence=[0.994 -11.8]  ExternalControl=on  NpNq=[1.3 2]  TimeConstants="[0  0  0  0]"  MinimumVoltage=0.7  Tfilter=-1  LoadFlowParameters=[4,0,0,0,0]
      settings: SourceProductBaseCode=PS
  Uniform Random Number : UniformRandomNumber  Minimum=-5e+1  Maximum=5e+1  Seed=1e+1  SampleTime=0.1
  A : PMIOPort  Side=Left
  B : PMIOPort  Port=2  Side=Left
  C : PMIOPort  Port=3  Side=Left
  Out1 : Outport
  m : Outport  Port=2
  wires:
  Mux2/1 -> Three-Phase Dynamic Load2/1
  Uniform Random Number/1 -> Matrix Multiply4/2
  Matrix Multiply4/1 -> Out1/1
  In3/1 -> Sum5/2
  Constant/1 -> Matrix Multiply4/1
  In1/1 -> Sum5/1
  Sum5/1 -> Mux2/1
  In4/1 -> Mux2/2
  Three-Phase Dynamic Load2/1 -> m/1
  connections:
  Three-Phase Dynamic Load2/LConn3 -- C/RConn1
  Three-Phase Dynamic Load2/LConn1 -- A/RConn1
  Three-Phase Dynamic Load2/LConn2 -- B/RConn1

== system FDIA_21_TRAINING/Subsystem1/Subsystem ==
  cte1 : Constant
  cte2 : Constant  Value=2
  cte3 : Constant  Value=0
  Generic : Outport  VectorParamsAs1DForOutWhenUnconnected=off
  Multiband : Outport  Port=2  VectorParamsAs1DForOutWhenUnconnected=off
  No PSS : Outport  Port=3  VectorParamsAs1DForOutWhenUnconnected=off
  wires:
  cte1/1 -> Generic/1
  cte2/1 -> Multiband/1
  cte3/1 -> No PSS/1

== system FDIA_21_TRAINING/Subsystem1/Subsystem1 ==
  Constant : Constant
  Constant16 : Constant  Value=11304000  SampleTime=-1
  Constant17 : Constant  Value=0
  Matrix Multiply5 : Product  Multiplication=Matrix(*)
  Mux1 : Mux  Inputs=2
  Scope34 : Scope
  Sum4 : Sum  Inputs=|++
  Three-Phase Dynamic Load1 : spsThreePhaseDynamicLoadLib/Three-Phase Dynamic Load  NominalVoltage="[ (217684)*1  60 ]"  ActiveReactivePowers=[11304000 0]  PositiveSequence=[0.994 -11.8]  ExternalControl=on  NpNq=[1.3 2]  TimeConstants="[0  0  0  0]"  MinimumVoltage=0.7  Tfilter=-1  LoadFlowParameters=[4,0,0,0,0]
      settings: SourceProductBaseCode=PS
  Uniform Random Number : UniformRandomNumber  Minimum=-5e+1  Maximum=5e+1  Seed=1e+1  SampleTime=0.1
  A : PMIOPort  Side=Left
  B : PMIOPort  Port=2  Side=Left
  C : PMIOPort  Port=3  Side=Left
  Out1 : Outport
  m : Outport  Port=2
  wires:
  Constant17/1 -> Mux1/2
  Constant/1 -> Matrix Multiply5/1
  Matrix Multiply5/1 -> Out1/1, Scope34/1, Sum4/1
  Uniform Random Number/1 -> Matrix Multiply5/2
  Three-Phase Dynamic Load1/1 -> m/1
  Sum4/1 -> Mux1/1
  Constant16/1 -> Sum4/2
  Mux1/1 -> Three-Phase Dynamic Load1/1
  connections:
  Three-Phase Dynamic Load1/LConn1 -- A/RConn1
  Three-Phase Dynamic Load1/LConn2 -- B/RConn1
  Three-Phase Dynamic Load1/LConn3 -- C/RConn1

== system FDIA_21_TRAINING/Subsystem1/Tie-Line Power Flow Sensor ==
  Constant : Constant
  Constant14 : Constant  Value=11304000  SampleTime=-1
  Constant15 : Constant  Value=0
  Matrix Multiply3 : Product  Multiplication=Matrix(*)
  Mux : Mux  Inputs=2
  Scope10 : Scope
  Scope33 : Scope
  Sum3 : Sum  Inputs=|++
  Three-Phase Dynamic Load : spsThreePhaseDynamicLoadLib/Three-Phase Dynamic Load  NominalVoltage="[ (217684)*1  60 ]"  ActiveReactivePowers=[11304000 0]  PositiveSequence=[0.994 -11.8]  ExternalControl=on  NpNq=[1.3 2]  TimeConstants="[0  0  0  0]"  MinimumVoltage=0.7  Tfilter=-1  LoadFlowParameters=[4,0,0,0,0]
      settings: SourceProductBaseCode=PS
  Uniform Random Number : UniformRandomNumber  Minimum=-5e+1  Maximum=5e+1  Seed=1e+1  SampleTime=0.1
  A : PMIOPort  Side=Left
  B : PMIOPort  Port=2  Side=Left
  C : PMIOPort  Port=3  Side=Left
  p1 : Outport
  m : Outport  Port=2
  wires:
  Mux/1 -> Three-Phase Dynamic Load/1
  Constant14/1 -> Sum3/2
  Sum3/1 -> Mux/1, Scope10/1
  Uniform Random Number/1 -> Matrix Multiply3/2
  Three-Phase Dynamic Load/1 -> m/1
  Matrix Multiply3/1 -> Scope33/1, p1/1, Sum3/1
  Constant15/1 -> Mux/2
  Constant/1 -> Matrix Multiply3/1
  connections:
  Three-Phase Dynamic Load/LConn2 -- B/RConn1
  Three-Phase Dynamic Load/LConn1 -- A/RConn1
  Three-Phase Dynamic Load/LConn3 -- C/RConn1

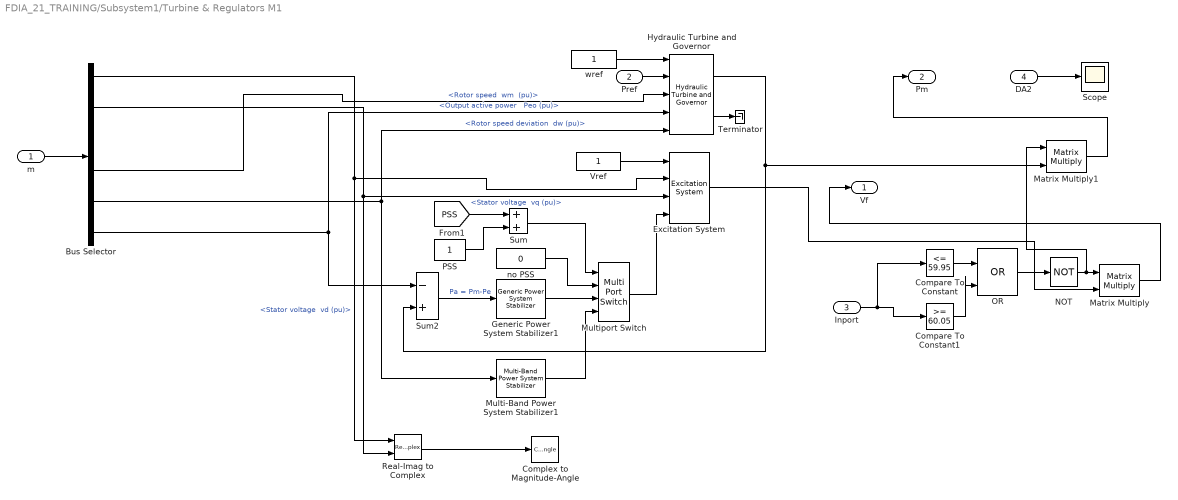
== system FDIA_21_TRAINING/Subsystem1/Turbine & Regulators M1 ==
  m : Inport
  Pref : Inport  Port=2
  Inport : Inport  Port=3
  DA2 : Inport  Port=4
  Bus Selector : BusSelector  OutputSignals="dq0 components.Stator voltage  vd (pu),dq0 components.Stator voltage  vq (pu),Mechanical.Rotor angle deviation  d_theta (rad),Mechanical.Rotor speed  wm  (pu),Mechanical.Rotor speed deviation  dw (pu),Output active power   Peo (pu)"
  Compare To Constant : simulink/Logic and Bit Operations/Compare To Constant  relop=<=  const=59.95  OutDataTypeStr=boolean
  Compare To Constant1 : simulink/Logic and Bit Operations/Compare To Constant  relop=>=  const=60.05  OutDataTypeStr=boolean
  Complex to Magnitude-Angle : ComplexToMagnitudeAngle  Output=Magnitude
  Excitation System : spsExcitationSystemLib/Excitation System  tr=20e-3  reg=[ 200, 0.001 ]  exc=[ 1, 0 ]  tgr=[ 0, 0 ]  damp=[ 0.001, 0.1 ]  sat=[ 0, 0 ]  lim="[ 0,  7, 0 ]"  v0=[1 2.8855]
      settings: SourceProductBaseCode=PS
  Generic Power System Stabilizer1 : spsGenericPowerSystemStabilizerLib/Generic Power System Stabilizer  Tsensor=15e-3  K=2  Twashout=0.7  Tleadlag1="[60e-3  0.5]"  Tleadlag2=[0 0]  VSlimits=[-0.15 0.15]  Vinit=0  Plot_On=off  MagdB_On=on  FreqRange=logspace(-2,2,500)
      settings: SourceProductBaseCode=PS
  Hydraulic Turbine and Governor : spsHydraulicTurbineandGovernorLib/Hydraulic Turbine and Governor  sm="[ 10/3  0.07 ]"  gate="[  0.01  0.97518  -0.1  0.1 ]"  reg="[  0.05  1.163  0.105  0  0.01  ]"  hyd="[  0  2.67  ]"  dref=0  po=1.0094
      settings: SourceProductBaseCode=PS
  Matrix Multiply : Product  Multiplication=Matrix(*)
  Matrix Multiply1 : Product  Multiplication=Matrix(*)
  Multi-Band Power System Stabilizer1 : spsMultiBandPowerSystemStabilizerLib/Multi-Band Power System Stabilizer  OperationMode=Simplified settings  Kg=1.0  GL=[0.2 20]  GI=[0.9 25]  GH=[12.0 145]  GLd=[66 66 9.4]  TcLF=[1.667 2 0 0 0 0 2 2.4 0 0 0 0 1 1]  GId=[66 66 47.6]  TcIF=[1 1 0.25 0.3 0 0 1 1 0.3 0.36 0 0 0 0]  GHd=[66 66 233]  TcHF="[0.01 0.012 0 0 0 0  0.012 0.0144 0 0 0 0 1 1]"  LIM=[.075 .15 .15 .15]  Plot_On=off  MagdB_On=off  FreqRange=logspace(-2,2,500)
      settings: SourceProductBaseCode=PS
  Multiport Switch : MultiPortSwitch  SaturateOnIntegerOverflow=on
  NOT : Logic  Operator=NOT  IconShape=distinctive  AllPortsSameDT=off  OutDataTypeStr=boolean
  OR : Logic  Operator=OR  IconShape=distinctive  AllPortsSameDT=off  OutDataTypeStr=boolean
  PSS : Constant
  Real-Imag to Complex : RealImagToComplex
  Scope : Scope
  Sum : Sum  SaturateOnIntegerOverflow=on
  Sum2 : Sum  Inputs=-+  InputSameDT=on  SaturateOnIntegerOverflow=on  OutDataTypeStr=Inherit: Same as first input
  Terminator : Terminator
  Vref : Constant
  no PSS : Constant  Value=0
  wref : Constant
  Vf : Outport  InitialOutput=0  VectorParamsAs1DForOutWhenUnconnected=off
  Pm : Outport  Port=2  InitialOutput=0  VectorParamsAs1DForOutWhenUnconnected=off
  wires:
  PSS/1 -> Sum/2
  [PSS] -> Sum/1
  Real-Imag to Complex/1 -> Complex to Magnitude-Angle/1
  Hydraulic Turbine and Governor/2 -> Terminator/1
  Vref/1 -> Excitation System/1
  m/1 -> Bus Selector/1
  Bus Selector/5 -> Multi-Band Power System Stabilizer1/1, Hydraulic Turbine and Governor/5  "<Rotor speed deviation  dw (pu)>"
  Bus Selector/6 -> Hydraulic Turbine and Governor/4, Sum2/1  "<Output active power   Peo (pu)>"
  Bus Selector/4 -> Hydraulic Turbine and Governor/3  "<Rotor speed  wm  (pu)>"
  Pref/1 -> Hydraulic Turbine and Governor/2
  wref/1 -> Hydraulic Turbine and Governor/1
  Hydraulic Turbine and Governor/1 -> Matrix Multiply1/2, Sum2/2
  Bus Selector/2 -> Excitation System/3, Real-Imag to Complex/2  "<Stator voltage  vq (pu)>"
  Excitation System/1 -> Matrix Multiply/2
  Bus Selector/1 -> Excitation System/2, Real-Imag to Complex/1  "<Stator voltage  vd (pu)>"
  Sum2/1 -> Generic Power System Stabilizer1/1  "Pa = Pm-Pe"
  Generic Power System Stabilizer1/1 -> Multiport Switch/3
  Multi-Band Power System Stabilizer1/1 -> Multiport Switch/4
  no PSS/1 -> Multiport Switch/2
  Sum/1 -> Multiport Switch/1
  Multiport Switch/1 -> Excitation System/4
  Inport/1 -> Compare To Constant/1, Compare To Constant1/1
  Compare To Constant1/1 -> OR/2
  OR/1 -> NOT/1
  Compare To Constant/1 -> OR/1
  NOT/1 -> Matrix Multiply1/1, Matrix Multiply/1
  Matrix Multiply/1 -> Vf/1
  Matrix Multiply1/1 -> Pm/1
  DA2/1 -> Scope/1

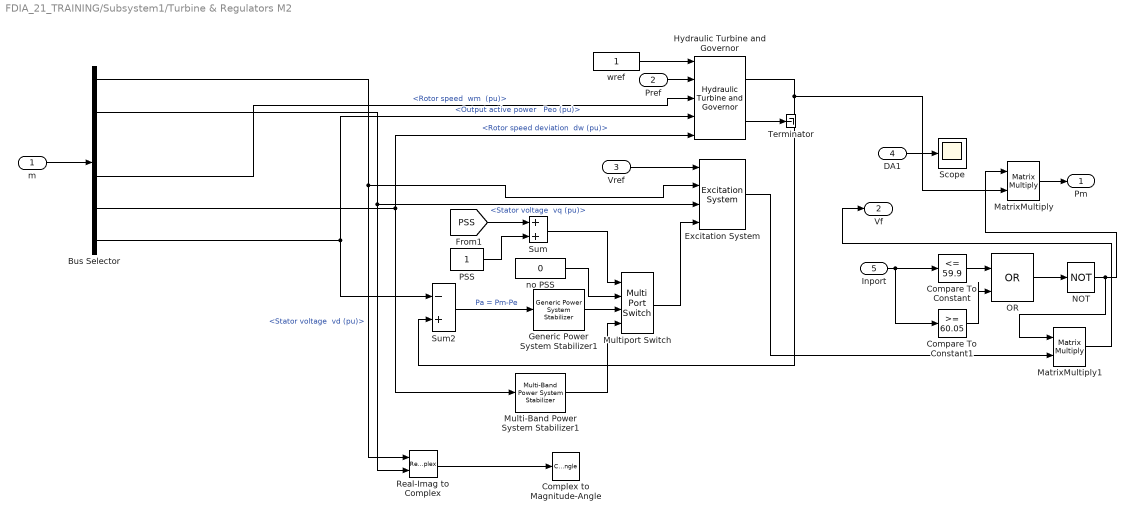
== system FDIA_21_TRAINING/Subsystem1/Turbine & Regulators M2 ==
  m : Inport
  Pref : Inport  Port=2
  Vref : Inport  Port=3
  DA1 : Inport  Port=4
  Inport : Inport  Port=5
  Bus Selector : BusSelector  OutputSignals="dq0 components.Stator voltage  vd (pu),dq0 components.Stator voltage  vq (pu),Mechanical.Rotor angle deviation  d_theta (rad),Mechanical.Rotor speed  wm  (pu),Mechanical.Rotor speed deviation  dw (pu),Output active power   Peo (pu)"
  Compare To Constant : simulink/Logic and Bit Operations/Compare To Constant  relop=<=  const=59.9  OutDataTypeStr=boolean
  Compare To Constant1 : simulink/Logic and Bit Operations/Compare To Constant  relop=>=  const=60.05  OutDataTypeStr=boolean
  Complex to Magnitude-Angle : ComplexToMagnitudeAngle  Output=Magnitude
  Excitation System : spsExcitationSystemLib/Excitation System  tr=20e-3  reg=[ 200, 0.001 ]  exc=[ 1, 0 ]  tgr=[ 0, 0 ]  damp=[ 0.001, 0.1 ]  sat=[ 0, 0 ]  lim="[ 0,  7, 0 ]"  v0=[1 2.4169]
      settings: SourceProductBaseCode=PS
  Generic Power System Stabilizer1 : spsGenericPowerSystemStabilizerLib/Generic Power System Stabilizer  Tsensor=15e-3  K=2  Twashout=0.7  Tleadlag1="[60e-3  0.5]"  Tleadlag2=[0 0]  VSlimits=[-0.15 0.15]  Vinit=0  Plot_On=off  MagdB_On=on  FreqRange=logspace(-2,2,500)
      settings: SourceProductBaseCode=PS
  Hydraulic Turbine and Governor : spsHydraulicTurbineandGovernorLib/Hydraulic Turbine and Governor  sm="[ 10/3  0.07 ]"  gate="[  0.01  0.97518  -0.1  0.1 ]"  reg="[  0.05  1.163  0.105  0  0.01  ]"  hyd="[  0  2.67  ]"  dref=0  po=1.0094
      settings: SourceProductBaseCode=PS
  MatrixMultiply : Product  Multiplication=Matrix(*)
  MatrixMultiply1 : Product  Multiplication=Matrix(*)
  Multi-Band Power System Stabilizer1 : spsMultiBandPowerSystemStabilizerLib/Multi-Band Power System Stabilizer  OperationMode=Simplified settings  Kg=1.0  GL=[0.025 5]  GI=[0.8 25]  GH=[12.0 145]  GLd=[66 66 9.4]  TcLF=[1.667 2 0 0 0 0 2 2.4 0 0 0 0 1 1]  GId=[66 66 47.6]  TcIF=[1 1 0.25 0.3 0 0 1 1 0.3 0.36 0 0 0 0]  GHd=[66 66 233]  TcHF="[0.01 0.012 0 0 0 0  0.012 0.0144 0 0 0 0 1 1]"  LIM=[.075 .15 .15 .15]  Plot_On=off  MagdB_On=off  FreqRange=logspace(-2,2,500)
      settings: SourceProductBaseCode=PS
  Multiport Switch : MultiPortSwitch  SaturateOnIntegerOverflow=on
  NOT : Logic  Operator=NOT  IconShape=distinctive  AllPortsSameDT=off  OutDataTypeStr=boolean
  OR : Logic  Operator=OR  IconShape=distinctive  AllPortsSameDT=off  OutDataTypeStr=boolean
  PSS : Constant
  Real-Imag to Complex : RealImagToComplex
  Scope : Scope
  Sum : Sum  SaturateOnIntegerOverflow=on
  Sum2 : Sum  Inputs=-+  InputSameDT=on  SaturateOnIntegerOverflow=on  OutDataTypeStr=Inherit: Same as first input
  Terminator : Terminator
  no PSS : Constant  Value=0
  wref : Constant
  Pm : Outport  InitialOutput=0  VectorParamsAs1DForOutWhenUnconnected=off
  Vf : Outport  Port=2  InitialOutput=0  VectorParamsAs1DForOutWhenUnconnected=off
  wires:
  PSS/1 -> Sum/2
  [PSS] -> Sum/1
  Real-Imag to Complex/1 -> Complex to Magnitude-Angle/1
  Hydraulic Turbine and Governor/2 -> Terminator/1
  Vref/1 -> Excitation System/1
  m/1 -> Bus Selector/1
  Bus Selector/5 -> Hydraulic Turbine and Governor/5, Multi-Band Power System Stabilizer1/1  "<Rotor speed deviation  dw (pu)>"
  Bus Selector/6 -> Hydraulic Turbine and Governor/4, Sum2/1  "<Output active power   Peo (pu)>"
  Bus Selector/4 -> Hydraulic Turbine and Governor/3  "<Rotor speed  wm  (pu)>"
  Pref/1 -> Hydraulic Turbine and Governor/2
  wref/1 -> Hydraulic Turbine and Governor/1
  Hydraulic Turbine and Governor/1 -> MatrixMultiply/2, Sum2/2
  Bus Selector/2 -> Excitation System/3, Real-Imag to Complex/2  "<Stator voltage  vq (pu)>"
  Excitation System/1 -> MatrixMultiply1/2
  Bus Selector/1 -> Excitation System/2, Real-Imag to Complex/1  "<Stator voltage  vd (pu)>"
  Sum2/1 -> Generic Power System Stabilizer1/1  "Pa = Pm-Pe"
  Generic Power System Stabilizer1/1 -> Multiport Switch/3
  Multi-Band Power System Stabilizer1/1 -> Multiport Switch/4
  no PSS/1 -> Multiport Switch/2
  Sum/1 -> Multiport Switch/1
  Multiport Switch/1 -> Excitation System/4
  DA1/1 -> Scope/1
  Inport/1 -> Compare To Constant1/1, Compare To Constant/1
  Compare To Constant/1 -> OR/1
  Compare To Constant1/1 -> OR/2
  OR/1 -> NOT/1
  NOT/1 -> MatrixMultiply1/1, MatrixMultiply/1
  MatrixMultiply/1 -> Pm/1
  MatrixMultiply1/1 -> Vf/1

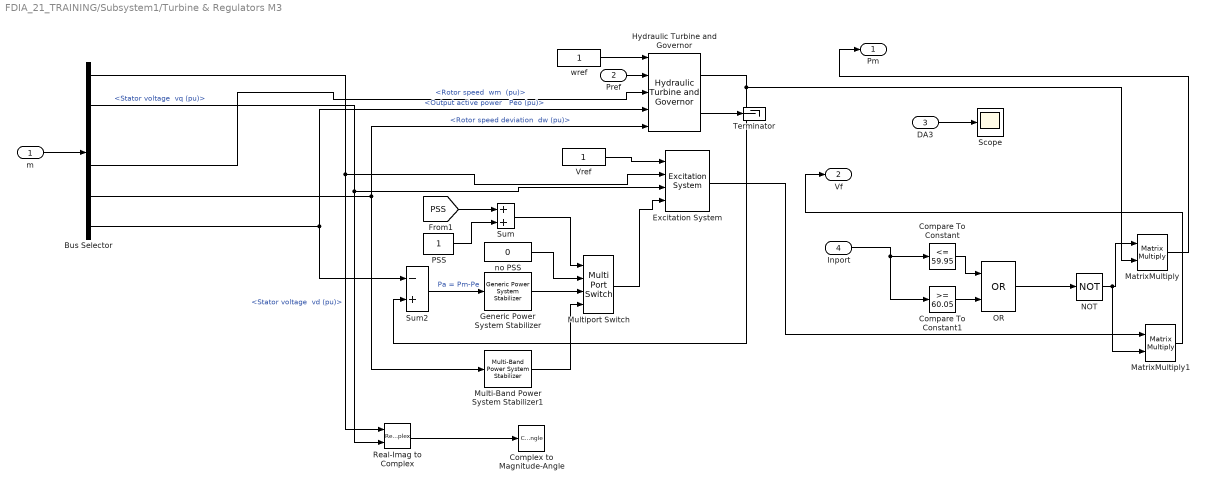
== system FDIA_21_TRAINING/Subsystem1/Turbine & Regulators M3 ==
  m : Inport
  Pref : Inport  Port=2
  DA3 : Inport  Port=3
  Inport : Inport  Port=4
  Bus Selector : BusSelector  OutputSignals="dq0 components.Stator voltage  vd (pu),dq0 components.Stator voltage  vq (pu),Mechanical.Rotor angle deviation  d_theta (rad),Mechanical.Rotor speed  wm  (pu),Mechanical.Rotor speed deviation  dw (pu),Output active power   Peo (pu)"
  Compare To Constant : simulink/Logic and Bit Operations/Compare To Constant  relop=<=  const=59.95  OutDataTypeStr=boolean
  Compare To Constant1 : simulink/Logic and Bit Operations/Compare To Constant  relop=>=  const=60.05  OutDataTypeStr=boolean
  Complex to Magnitude-Angle : ComplexToMagnitudeAngle  Output=Magnitude
  Excitation System : spsExcitationSystemLib/Excitation System  tr=20e-3  reg=[200, 0.001 ]  exc=[ 1, 0 ]  tgr=[ 0, 0 ]  damp=[ 0.001, 0.1 ]  sat=[ 0, 0 ]  lim="[ 0,  7, 0 ]"  v0=[1.0117 1.7297]
      settings: SourceProductBaseCode=PS
  Generic Power System Stabilizer : spsGenericPowerSystemStabilizerLib/Generic Power System Stabilizer  Tsensor=30e-3  K=20  Twashout=2  Tleadlag1=[50e-3 20e-3]  Tleadlag2=[3 5.4]  VSlimits=[-0.15 0.15]  Vinit=0  Plot_On=off  MagdB_On=on  FreqRange=logspace(-2,2,500)
      settings: SourceProductBaseCode=PS
  Hydraulic Turbine and Governor : spsHydraulicTurbineandGovernorLib/Hydraulic Turbine and Governor  sm="[ 10/3  0.07 ]"  gate="[  0.01  0.97518  -0.1  0.1 ]"  reg="[  0.05  1.163  0.105  0  0.01  ]"  hyd="[  0  2.67  ]"  dref=0  po=0.010371
      settings: SourceProductBaseCode=PS
  MatrixMultiply : Product  Multiplication=Matrix(*)
  MatrixMultiply1 : Product  Multiplication=Matrix(*)
  Multi-Band Power System Stabilizer1 : spsMultiBandPowerSystemStabilizerLib/Multi-Band Power System Stabilizer  OperationMode=Simplified settings  Kg=1.0  GL=[0.2 20]  GI=[0.9 25]  GH=[12.0 145]  GLd=[66 66 9.4]  TcLF=[1.667 2 0 0 0 0 2 2.4 0 0 0 0 1 1]  GId=[66 66 47.6]  TcIF=[1 1 0.25 0.3 0 0 1 1 0.3 0.36 0 0 0 0]  GHd=[66 66 233]  TcHF="[0.01 0.012 0 0 0 0  0.012 0.0144 0 0 0 0 1 1]"  LIM=[.075 .15 .15 .15]  Plot_On=off  MagdB_On=off  FreqRange=logspace(-2,2,500)
      settings: SourceProductBaseCode=PS
  Multiport Switch : MultiPortSwitch  SaturateOnIntegerOverflow=on
  NOT : Logic  Operator=NOT  IconShape=distinctive  AllPortsSameDT=off  OutDataTypeStr=boolean
  OR : Logic  Operator=OR  IconShape=distinctive  AllPortsSameDT=off  OutDataTypeStr=boolean
  PSS : Constant
  Real-Imag to Complex : RealImagToComplex
  Scope : Scope
  Sum : Sum  SaturateOnIntegerOverflow=on
  Sum2 : Sum  Inputs=-+  InputSameDT=on  SaturateOnIntegerOverflow=on  OutDataTypeStr=Inherit: Same as first input
  Terminator : Terminator
  Vref : Constant
  no PSS : Constant  Value=0
  wref : Constant
  Pm : Outport  InitialOutput=0  VectorParamsAs1DForOutWhenUnconnected=off
  Vf : Outport  Port=2  InitialOutput=0  VectorParamsAs1DForOutWhenUnconnected=off
  wires:
  PSS/1 -> Sum/2
  [PSS] -> Sum/1
  Real-Imag to Complex/1 -> Complex to Magnitude-Angle/1
  Hydraulic Turbine and Governor/2 -> Terminator/1
  Vref/1 -> Excitation System/1
  m/1 -> Bus Selector/1
  Bus Selector/5 -> Hydraulic Turbine and Governor/5, Multi-Band Power System Stabilizer1/1  "<Rotor speed deviation  dw (pu)>"
  Bus Selector/6 -> Hydraulic Turbine and Governor/4, Sum2/1  "<Output active power   Peo (pu)>"
  Bus Selector/4 -> Hydraulic Turbine and Governor/3  "<Rotor speed  wm  (pu)>"
  Pref/1 -> Hydraulic Turbine and Governor/2
  wref/1 -> Hydraulic Turbine and Governor/1
  Hydraulic Turbine and Governor/1 -> MatrixMultiply/2, Sum2/2
  Bus Selector/2 -> Excitation System/3, Real-Imag to Complex/2  "<Stator voltage  vq (pu)>"
  Excitation System/1 -> MatrixMultiply1/1
  Bus Selector/1 -> Excitation System/2, Real-Imag to Complex/1  "<Stator voltage  vd (pu)>"
  Sum2/1 -> Generic Power System Stabilizer/1  "Pa = Pm-Pe"
  Generic Power System Stabilizer/1 -> Multiport Switch/3
  Multi-Band Power System Stabilizer1/1 -> Multiport Switch/4
  no PSS/1 -> Multiport Switch/2
  Sum/1 -> Multiport Switch/1
  Multiport Switch/1 -> Excitation System/4
  Inport/1 -> Compare To Constant1/1, Compare To Constant/1
  Compare To Constant/1 -> OR/1
  Compare To Constant1/1 -> OR/2
  OR/1 -> NOT/1
  NOT/1 -> MatrixMultiply1/2, MatrixMultiply/1
  DA3/1 -> Scope/1
  MatrixMultiply/1 -> Pm/1
  MatrixMultiply1/1 -> Vf/1

== matlab function FDIA_21_TRAINING/Subsystem1/MATLAB Function1 ==
  data: u input; y output
function y = fcn(u)

y = norm(u+2,"inf");

== matlab function FDIA_21_TRAINING/Subsystem1/MATLAB Function ==
  data: u input; y output
function y = fcn(u)

y = norm(u,"inf");

== matlab function FDIA_21_TRAINING/DEFENDER REWARD FUNCTION ==
  data: DAF1 input; DAF2 input; DAF3 input; REWARD_DEFENDER output; DAR input; DATHD input
function REWARD_DEFENDER = fcn(DAF1,DAF2,DAF3, DAR, DATHD)

REWARD_DEFENDER = 0.5.*(1-abs((DAF1-60)/0.5))+0.5.*(1-abs((DAF2-60)/0.5))+0.5.*(1-abs((DAF3-60)/0.5)) + 0.5.*(1-abs((DAR-4)/4)) + 0.5.*(1-abs((DATHD-10e4)/10e4));
end

== matlab function FDIA_21_TRAINING/Subsystem1/MATLAB Function2 ==
  data: u input; y output
function y = fcn(u)

y = norm(u+1,"inf");
